simulink subsystem "EngineBasic_refsub"  (R2020b)
settings: Solver=VariableStepAuto  StartTime=0.0  StopTime=10.0  RelTol=1e-3
undefined symbols (not defined in the file): engine
libraries: fl_lib x9, nesl_utility x2, sdl_lib x1
settings Model: Creator=isaacito  LastModifiedBy=isaacito

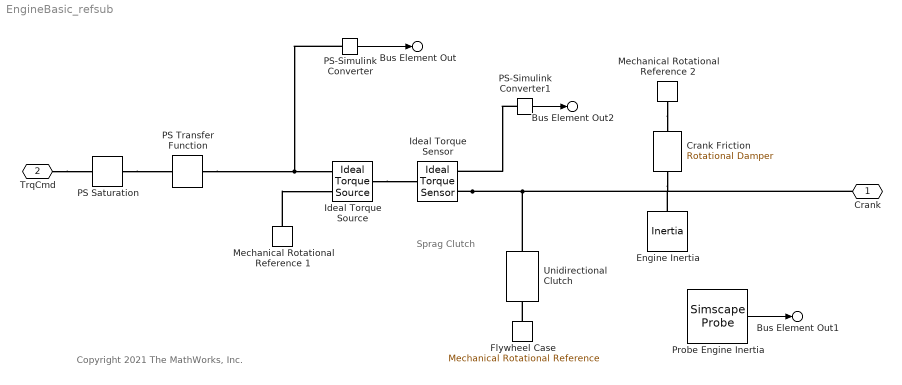
== system EngineBasic_refsub ==
  note: Sprag Clutch
  note: Copyright 2021 The MathWorks, Inc.
  Crank Friction : fl_lib/Mechanical/Rotational Elements/Rotational Damper  D=engine.damping_Nm_per_rpm N*m/rpm  w_specify=off  w_priority=None  w=0 rad/s  w_nominal_specify=off  w_nominal_unit=rad/s  w_nominal_value=1  t_specify=off  t_priority=None  t=0 N*m  t_nominal_specify=off  t_nominal_unit=N*m  t_nominal_value=1
  Engine Inertia : fl_lib/Mechanical/Rotational Elements/Inertia  inertia=engine.inertia_kg_m2 kg*m^2  num_ports=foundation.enum.numPorts2.one  w_specify=on  w_priority=None  w=initial.engine_speed_rpm rpm  w_nominal_specify=off  w_nominal_unit=rad/s  w_nominal_value=1  t_specify=off  t_priority=None  t=0 N*m  t_nominal_specify=off  t_nominal_unit=N*m  t_nominal_value=1
      settings: AttributesFormatString=|
      | %<inertia> (%<inertia_unit>)
      | %<w> (%<w_unit>)
      | Priority: %<w_priority>
  Flywheel Case : fl_lib/Mechanical/Rotational Elements/Mechanical Rotational Reference
  Ideal Torque Sensor : fl_lib/Mechanical/Mechanical Sensors/Ideal Torque Sensor
  Ideal Torque Source : fl_lib/Mechanical/Mechanical Sources/Ideal Torque Source
  Mechanical Rotational Reference 1 : fl_lib/Mechanical/Rotational Elements/Mechanical Rotational Reference
  Mechanical Rotational Reference 2 : fl_lib/Mechanical/Rotational Elements/Mechanical Rotational Reference
  PS Saturation : fl_lib/Physical Signals/Nonlinear Operators/PS Saturation  upper_limit=engine.trqMax_Nm N*m  lower_limit=0 N*m
      settings: AttributesFormatString=%<upper_limit> (%<upper_limit_unit>)  SourceProductBaseCode=SS
  PS Transfer Function : fl_lib/Physical Signals/Linear Operators/PS Transfer Function  transfer_function_type=foundation.enum.transfer_function_type.lag  T=engine.lag_s s  T1=2 s  T2=1 s  y0=initial.engine_torque_Nm N*m
      settings: SourceProductBaseCode=SS  InternalSimscapePortConfiguration="{\"Bottom\":[],\"Left\":[{\"id\":\"U\",\"label\":\"\",\"type\":\"input\"}],\"Right\":[{\"id\":\"Y\",\"label\":\"\",\"type\":\"output\"}],\"Top\":[]}"
      settings: AttributesFormatString=|
      | %<T> [%<T_unit>]
      | Initial: %<y0> [%<y0_unit>]
  PS-Simulink Converter : nesl_utility/PS-Simulink Converter  PhysicalDomain=network_engine_domain  SubClassName=ps_output  LeftPortType=input  RightPortType=output  PseudoPeriodic=off  Frequencies=[]  Unit=N*m  AffineConversion=off
  PS-Simulink Converter1 : nesl_utility/PS-Simulink Converter  PhysicalDomain=network_engine_domain  SubClassName=ps_output  LeftPortType=input  RightPortType=output  PseudoPeriodic=off  Frequencies=[]  Unit=inherit  AffineConversion=off
  Probe Engine Inertia : SimscapeProbe  BoundBlock=2  Variables={w}
  Unidirectional Clutch : sdl_lib/Clutches/Unidirectional Clutch  transmission_direction=2  initial_state_locked=sdl.enum.initial_lock.locked
      settings: SourceProductBaseCode=LD  InternalSimscapePortConfiguration="{\"Bottom\":[],\"Left\":[{\"id\":\"H\",\"label\":\"H\",\"type\":\"foundation.mechanical.rotational.rotational\"}],\"Right\":[{\"id\":\"R\",\"label\":\"R\",\"type\":\"foundation.mechanical.rotational.rotational\"}],\"Top\":[]}"
  Crank : PMIOPort  Side=Left
  TrqCmd : PMIOPort  Port=2  Side=Right
  Bus Element Out : Outport  PortName=Info  Element=TrqCmd
      settings: AttributesFormatString=%<Unit>
  Bus Element Out1 : Outport  PortName=Info  Element=Spd
      settings: AttributesFormatString=%<Unit>
  Bus Element Out2 : Outport  PortName=Info  Element=Trq
      settings: AttributesFormatString=%<Unit>
  wires:
  PS-Simulink Converter/1 -> Bus Element Out/1
  Probe Engine Inertia/1 -> Bus Element Out1/1
  PS-Simulink Converter1/1 -> Bus Element Out2/1
  connections:
  Ideal Torque Sensor/RConn1 -- Crank Friction/LConn1 -- Engine Inertia/LConn1 -- Crank/RConn1 -- Unidirectional Clutch/LConn1
  PS-Simulink Converter/LConn1 -- PS Transfer Function/RConn1 -- Ideal Torque Source/RConn1
  Mechanical Rotational Reference 1/LConn1 -- Ideal Torque Source/RConn2
  PS Saturation/RConn1 -- PS Transfer Function/LConn1
  TrqCmd/RConn1 -- PS Saturation/LConn1
  Mechanical Rotational Reference 2/LConn1 -- Crank Friction/RConn1
  Ideal Torque Source/LConn1 -- Ideal Torque Sensor/LConn1
  PS-Simulink Converter1/LConn1 -- Ideal Torque Sensor/RConn2
  Flywheel Case/LConn1 -- Unidirectional Clutch/RConn1
